simulink model "A18bpsk7"  (Simulink 9.1)
settings: Solver=FixedStepDiscrete  StartTime=0.0  StopTime=1000  RelTol=1e-3  EnableMultiTasking=on
undefined symbols (not defined in the file): j
libraries: dsp_blocks x6
settings Model: Creator=DSP_Lab  LastModifiedBy=Hayoung
settings DataIOCC: LimitDataPoints=on
settings OptimizationCC: ExpressionDepthLimit=2147483647
settings DebuggingCC: SolverPrmCheckMsg=warning  StateNameClashWarn=warning
settings GRTTargetCC: GeneratePreprocessorConditionals=Disable all  CombineOutputUpdateFcns=on  GRTInterface=off

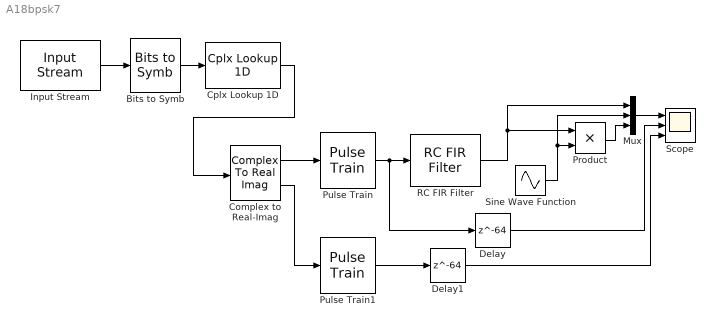
== system A18bpsk7 ==
  Bits to Symb : dsp_blocks/Conversions/Bits to Symb
  Complex to Real-Imag : ComplexToRealImag
  Cplx Lookup 1D : dsp_blocks/Conversions/Cplx Lookup 1D  table=[1 j -1 -j]
  Delay : Delay  DelayLength=64
  Delay1 : Delay  DelayLength=64
  Input Stream : dsp_blocks/Sources//Sinks/Input Stream  period=50  width=2  fname=rand.mat
  Mux : Mux  Inputs=3
  Product : Product  RndMeth=Zero
  Pulse Train : dsp_blocks/Conversions/Pulse Train  period=50
  Pulse Train1 : dsp_blocks/Conversions/Pulse Train  period=50
  RC FIR Filter : dsp_blocks/Filters/RC FIR Filter  period=50  beta=0.25  root=off  filt_len=128  win_type=on
  Scope : Scope  NumInputPorts=3
  Sine Wave Function : Sin  Frequency=2*pi*0.1  Phase=-pi/2  SampleTime=0
  wires:
  Input Stream/1 -> Bits to Symb/1
  Bits to Symb/1 -> Cplx Lookup 1D/1
  Pulse Train/1 -> RC FIR Filter/1, Delay/1
  RC FIR Filter/1 -> Mux/1, Product/1
  Sine Wave Function/1 -> Product/2, Mux/2
  Cplx Lookup 1D/1 -> Complex to Real-Imag/1
  Complex to Real-Imag/1 -> Pulse Train/1
  Complex to Real-Imag/2 -> Pulse Train1/1
  Pulse Train1/1 -> Delay1/1
  Delay/1 -> Scope/2
  Delay1/1 -> Scope/3
  Product/1 -> Mux/3
  Mux/1 -> Scope/1
